simulink model "example1"  (R2022b)
settings: Solver=VariableStepAuto  StartTime=0.0  StopTime=10.0  RelTol=1e-3
libraries: simulink x1
settings Model: Creator=Soliman Rabie  LastModifiedBy=Soliman Rabie

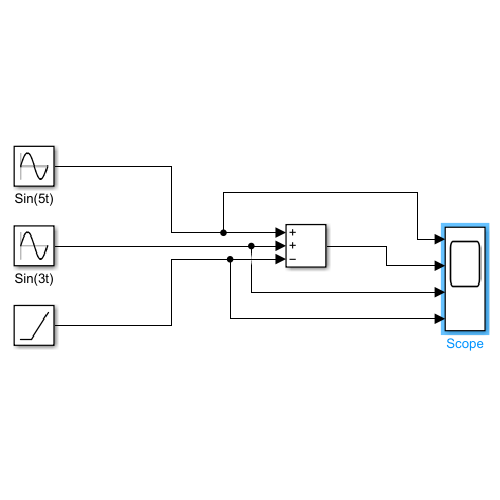
[thumbnail: Simulink's stored preview of the top-level diagram]
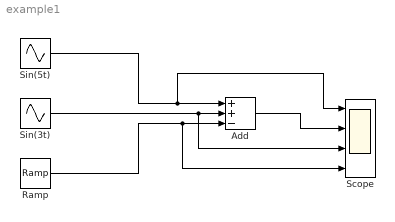
== system example1 ==
  Add : Sum  Inputs=++-
  Ramp : simulink/Sources/Ramp  slope=1  start=0  InitialOutput=0
  Scope : Scope  NumInputPorts=4
  Sin(3t) : Sin  Amplitude=3  SampleTime=0
  Sin(5t) : Sin  Amplitude=5  SampleTime=0
  wires:
  Sin(5t)/1 -> Scope/1, Add/1
  Sin(3t)/1 -> Scope/3, Add/2
  Ramp/1 -> Scope/4, Add/3
  Add/1 -> Scope/2
